simulink model "Pippo_sim"  (R2022b)
settings: Solver=ode1  StartTime=0.0  StopTime=inf  FixedStep=0.002  RelTol=1e-3  EnableMultiTasking=on
PostLoadFcn:
  | qc_set_target_type(getConfigSet(bdroot, 'QUARC Default Target Configuration'));
undefined symbols (not defined in the file or in its folder): HIL, qc_get_step_size
libraries: quarc_library x21, simulink_extras x7, simulink x6
settings Model: SimulationMode=external  ExtModeTrigDuration=10000  Creator=CFulford  LastModifiedBy=Utente
settings SolverCC: AlgebraicLoopSolver=TrustRegion  PositivePriorityOrder=on
settings DataIOCC: LimitDataPoints=on  SaveFormat=Array  SignalLoggingSaveFormat=ModelDataLogs  ReturnWorkspaceOutputs=off
settings OptimizationCC: ExpressionDepthLimit=2147483647  InitFltsAndDblsToZero=on
settings DebuggingCC: SaveWithParameterizedLinksMsg=none  UnderspecifiedInitializationDetection=Classic  MergeDetectMultiDrivingBlocksExec=none  SolverPrmCheckMsg=warning  MultiTaskDSMMsg=warning  MultiTaskCondExecSysMsg=none  FcnCallInpInsideContextMsg=warning  UnconnectedInputMsg=warning  UnconnectedOutputMsg=warning  UnconnectedLineMsg=warning  StateNameClashWarn=warning  SFUnexpectedBacktrackingDiag=warning  SFNoUnconditionalDefaultTransitionDiag=warning  SFExecutionAtInitializationDiag=none  SFMachineParentedDataDiag=warning  ArithmeticOperatorsInVariantConditions=warning
settings ModelReferenceCC: EnableRefExpFcnMdlSchedulingChecks=on  PropagateSignalLabelsOutOfModel=off
settings SFSimCC: SimUseLocalCustomCode=off  CustomCodeUndefinedFunction=UseInterfaceOnly
settings RTWCC: Description=QUARC Win64 Target Using Toolchain  SystemTargetFile=quarc_win64.tlc  TemplateMakefile=quarc_default_tmf  RTWUseLocalCustomCode=off  Toolchain=QUARC win64 | nmake (64-bit Windows)  BuildConfiguration=Faster Runs
settings CodeAppCC: StateflowObjectComments=on
settings STFCustomTargetCC: ConcurrentExecutionCompliant=on  GRTInterface=on  UseToolchainInfoCompliant=on  SystemTargetFile=quarc_win64.tlc
settings GRTTargetCC: TargetLangStandard=C89/C90 (ANSI)  ParMdlRefBuildCompliant=off  CompOptLevelCompliant=off  CombineOutputUpdateFcns=off  MatFileLogging=off  CPPClassGenCompliant=off  GRTInterface=on  ExtMode=on  ExtModeMexFile=quarc_comm
settings ConfigComp: CovMetricSettings=dw  CovSaveCumulativeToWorkspaceVar=on  CovSaveSingleToWorkspaceVar=on  CovExternalEMLEnable=off  CovSFcnEnable=off

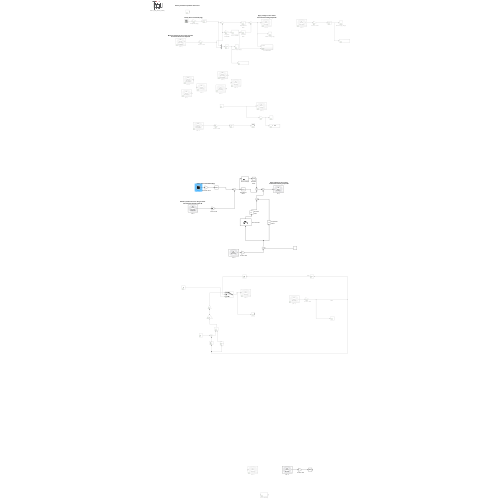
[thumbnail: Simulink's stored preview of the top-level diagram]
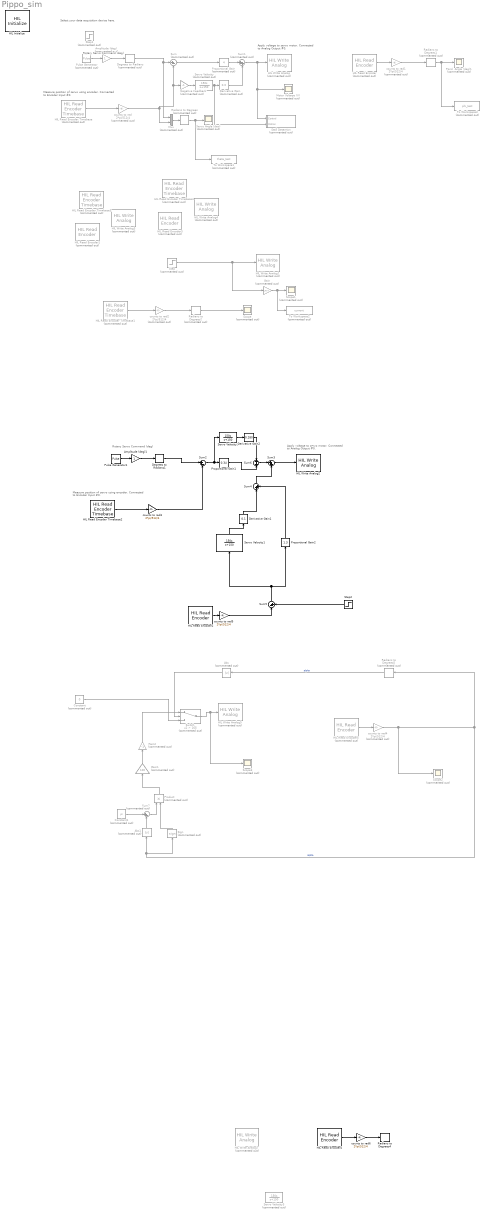
== system Pippo_sim ==
  note: Apply voltage to servo motor.
      | Connected to Analog Output #0.
  note: Measure position of servo using encoder.
      | Connected to Encoder Input #0.
  note: Select your data acquisition device here.
  note: Rotary Servo Command (deg)
  note: Measure position of servo using encoder.
      | Connected to Encoder Input #0.
  note: Rotary Servo Command (deg)
  note: Apply voltage to servo motor.
      | Connected to Analog Output #0.
  Abs : Abs  Commented=on  SaturateOnIntegerOverflow=off
  Abs1 : Abs  Commented=on  SaturateOnIntegerOverflow=off
  Amplitude (deg) : Gain  Commented=on
  Amplitude (deg)1 : Gain
  Constant : Constant  Commented=on  Value=0
  Constant1 : Constant  Commented=on  Value=pi
  Degrees to Radians : simulink_extras/Transformations/Degrees to Radians  Commented=on
  Degrees to Radians1 : simulink_extras/Transformations/Degrees to Radians
  Derivative Gain : simulink/Math Operations/Slider Gain  Commented=on  gain=0.0  low=0  high=0.5
  Derivative Gain1 : simulink/Math Operations/Slider Gain  gain=0.1  low=0  high=0.5
  Derivative Gain2 : simulink/Math Operations/Slider Gain  gain=0.280  low=0  high=0.5
  Gain : Gain  Commented=on  Gain=1/8.4
  Gain1 : Gain  Commented=on  Gain=100
  Gain2 : Gain  Commented=on  Gain=-1
  HIL Initialize : quarc_library/Data Acquisition/Generic/Configuration/HIL Initialize  Priority=-99  object_name=HIL-1  board_type=qube_servo2_usb  board_number=0  board_options=""  exclusive=off  active=off  hardware_clocks=[0]  clock_modes=[]  initial_clock_frequencies=[]  set_clock_params_at_start=off  set_clock_params_at_switch_in=off  set_clock_frequencies_at_start=off  set_clock_frequencies_at_switch_in=off  analog_input_channels=[0]  analog_input_configurations=[]  analog_input_maximums=3  analog_input_minimums=-3  set_analog_input_params_at_start=off  set_analog_input_params_at_switch_in=off  analog_output_channels=[0]  analog_output_maximums=15  analog_output_minimums=-15  initial_analog_outputs=[0]  final_analog_outputs=[0]  watchdog_analog_outputs=0  set_analog_output_params_at_start=off  set_analog_output_params_at_switch_in=off  set_analog_outputs_at_start=on  set_analog_outputs_at_switch_in=off  set_analog_outputs_at_terminate=on  set_analog_outputs_at_switch_out=off  set_analog_outputs_on_watchdog=on  digital_input_channels=[]  digital_output_channels=[0]  digital_output_configuration=[]  initial_digital_outputs=[1]  final_digital_outputs=[0]  watchdog_digital_outputs=[0]  set_digital_output_params_at_start=off  set_digital_output_params_at_switch_in=off  set_digital_outputs_at_start=on  set_digital_outputs_at_switch_in=off  set_digital_outputs_at_terminate=on  set_digital_outputs_at_switch_out=off  set_digital_outputs_on_watchdog=on  encoder_channels=[0:1]  quadrature=[4]  encoder_filter_frequency=[]  initial_encoder_counts=[0]  set_encoder_params_at_start=off  set_encoder_params_at_switch_in=off  set_encoder_counts_at_start=on  set_encoder_counts_at_switch_in=off  pwm_channels=[]  pwm_modes=[]  pwm_frequency=[]  pwm_configuration=[]  pwm_alignment=[]  pwm_polarity=[]  pwm_leading_deadband=[]  pwm_trailing_deadband=[]  initial_pwm_outputs=[]  final_pwm_outputs=[]  watchdog_pwm_outputs=[]  set_pwm_params_at_start=off  set_pwm_params_at_switch_in=off  set_pwm_outputs_at_start=off  set_pwm_outputs_at_switch_in=off  set_pwm_outputs_at_terminate=off  set_pwm_outputs_at_switch_out=off  set_pwm_outputs_on_watchdog=off  other_output_channels=[11000:11002]  initial_other_outputs=[0 1 0]  final_other_outputs=[1 0 0]  watchdog_other_outputs=[0 0 1]  set_other_outputs_at_start=on  set_other_outputs_at_switch_in=off  set_other_outputs_at_terminate=on  set_other_outputs_at_switch_out=off  set_other_outputs_on_watchdog=on
  HIL Read Encoder{,1,3,5} (4 alike) : quarc_library/Data Acquisition/Generic/Immediate I//O/HIL Read Encoder  Commented=on  object_name=HIL-1  channels=[1]  sample_time=qc_get_step_size  active=on  vector_output=off  data_type_mode=Inherit via back propagation  data_type=double
  HIL Read Encoder Timebase{,1,3..4} (4 alike) : quarc_library/Data Acquisition/Generic/Timebases/HIL Read Encoder Timebase  Commented=on  object_name=HIL-1  clock=0  channels=0  active=on  vector_output=off  data_type_mode=Inherit via back propagation  data_type=double  overflow_mode=Error on overflow  samples_in_buffer=max(ceil(1/qc_get_step_size), 1)
  HIL Read Encoder Timebase2 : quarc_library/Data Acquisition/Generic/Timebases/HIL Read Encoder Timebase  object_name=HIL-1  clock=0  channels=0  active=on  vector_output=off  data_type_mode=Inherit via back propagation  data_type=double  overflow_mode=Error on overflow  samples_in_buffer=max(ceil(1/qc_get_step_size), 1)
  HIL Read Encoder2 : quarc_library/Data Acquisition/Generic/Immediate I//O/HIL Read Encoder  object_name=HIL-1  channels=[1]  sample_time=qc_get_step_size  active=on  vector_output=off  data_type_mode=Inherit via back propagation  data_type=double
  HIL Read Encoder4 : quarc_library/Data Acquisition/Generic/Immediate I//O/HIL Read Encoder  object_name=HIL-1  channels=[1]  sample_time=qc_get_step_size  active=on  vector_output=off  data_type_mode=Inherit via back propagation  data_type=double
  HIL Write Analog{,1,3..5,7} (6 alike) : quarc_library/Data Acquisition/Generic/Immediate I//O/HIL Write Analog  Commented=on  object_name=HIL-1  channels=0  sample_time=-1  active=off  vector_input=off
  HIL Write Analog2 : quarc_library/Data Acquisition/Generic/Immediate I//O/HIL Write Analog  object_name=HIL-1  channels=0  sample_time=-1  active=off  vector_input=off
  Motor Voltage (V) : Scope  Commented=on
  Mux : Mux  Commented=on  Inputs=2
  Negative Feedback : Gain  Commented=on  Gain=-1
  Pend  Angle (deg)1 : Scope  Commented=on
  Product : Product  Commented=on
  Proportional Gain : simulink/Math Operations/Slider Gain  Commented=on  gain=4  low=0  high=10
  Proportional Gain1 : simulink/Math Operations/Slider Gain  gain=0.34  low=0  high=10
  Proportional Gain2 : simulink/Math Operations/Slider Gain  gain=1.3  low=0  high=10
  Pulse Generator : DiscretePulseGenerator  Commented=on  PulseType=Time based  Amplitude=90  Period=10  PulseWidth=50
  Pulse Generator1 : DiscretePulseGenerator  PulseType=Time based  Amplitude=0  Period=10  PulseWidth=50
  Radians to Degrees{,1..2,5} (4 alike) : simulink_extras/Transformations/Radians to Degrees  Commented=on
  Radians to Degrees4 : simulink_extras/Transformations/Radians to Degrees
  Scope{,1..3} (4 alike) : Scope  Commented=on
  Servo Angle (deg) : Scope  Commented=on
  Servo Velocity : TransferFcn  Commented=on  Numerator=[150 0]  Denominator=[1 150]
  Servo Velocity1 : TransferFcn  Numerator=[150 0]  Denominator=[1 150]
  Servo Velocity2 : TransferFcn  Numerator=[150 0]  Denominator=[1 150]
  Servo Velocity3 : TransferFcn  Commented=on  Numerator=[150 0]  Denominator=[1 150]
  Sign : Signum  Commented=on
  Stall Detection : Subsystem  Commented=on
  Step : Step  Commented=on  SampleTime=0
  Step1 : Step  Commented=on  After=45  SampleTime=0
  Step2 : Step  Time=0  After=0  SampleTime=0
  Sum : Sum  Commented=on  Inputs=|+-
  Sum1 : Sum  Commented=on  Inputs=|++
  Sum2 : Sum  Inputs=|+-
  Sum3 : Sum  Inputs=|++
  Sum4 : Sum  Inputs=|++
  Sum5 : Sum  Inputs=|-+
  Sum6 : Sum
  Sum7 : Sum  Commented=on  Inputs=|+-
  Switch : Switch  Commented=on  Criteria=u2 > Threshold  Threshold=165  SaturateOnIntegerOverflow=off  InputSameDT=off
  To Workspace1 : ToWorkspace  Commented=on  VariableName=theta_test  SaveFormat=Structure With Time  SampleTime=-1
  To Workspace2 : ToWorkspace  Commented=on  VariableName=current  SaveFormat=Structure With Time  SampleTime=-1
  To Workspace3 : ToWorkspace  Commented=on  VariableName=phi_test  SaveFormat=Structure With Time  SampleTime=-1
  counts to rad{,1..2,4} (4 alike) : Gain  Commented=on  Gain=2*pi/512/4
  counts to rad3 : Gain  Gain=2*pi/512/4
  counts to rad5 : Gain  Gain=2*pi/512/4
  counts to rad6 : Gain  Gain=2*pi/512/4
  wires:
  Sum1/1 -> HIL Write Analog/1, Stall Detection/1(Control), Motor Voltage (V)/1
  Sum/1 -> Proportional Gain/1
  counts to rad/1 -> Sum/2, Negative Feedback/1, Mux/2
  Proportional Gain/1 -> Sum1/1
  Servo Velocity/1 -> Stall Detection/2(Motion), Derivative Gain/1
  Derivative Gain/1 -> Sum1/2
  Degrees to Radians/1 -> Mux/1, Sum/1
  Negative Feedback/1 -> Servo Velocity/1
  Mux/1 -> Radians to Degrees/1
  Radians to Degrees/1 -> To Workspace1/1, Servo Angle (deg)/1
  HIL Read Encoder/1 -> counts to rad1/1
  Radians to Degrees1/1 -> To Workspace3/1, Pend  Angle (deg)1/1
  counts to rad1/1 -> Radians to Degrees1/1
  Amplitude (deg)/1 -> Degrees to Radians/1
  Pulse Generator/1 -> Amplitude (deg)/1
  HIL Read Encoder Timebase/1 -> counts to rad/1
  Step/1 -> Gain/1, HIL Write Analog1/1
  HIL Read Encoder Timebase1/1 -> counts to rad2/1
  counts to rad2/1 -> Radians to Degrees2/1
  Gain/1 -> To Workspace2/1, Scope1/1
  Radians to Degrees2/1 -> Scope/1
  Pulse Generator1/1 -> Amplitude (deg)1/1
  Amplitude (deg)1/1 -> Degrees to Radians1/1
  Proportional Gain1/1 -> Sum6/2
  Sum3/1 -> HIL Write Analog2/1
  counts to rad3/1 -> Sum2/2
  HIL Read Encoder Timebase2/1 -> counts to rad3/1
  Sum5/1 -> Servo Velocity1/1, Proportional Gain2/1
  HIL Read Encoder2/1 -> counts to rad5/1
  Proportional Gain2/1 -> Sum4/2
  Servo Velocity1/1 -> Derivative Gain1/1
  Derivative Gain1/1 -> Sum4/1
  counts to rad5/1 -> Sum5/1
  Step2/1 -> Sum5/2
  Degrees to Radians1/1 -> Sum2/1
  Sum2/1 -> Servo Velocity2/1, Proportional Gain1/1
  Servo Velocity2/1 -> Derivative Gain2/1
  Sum6/1 -> Sum3/1
  Sum4/1 -> Sum3/2
  Derivative Gain2/1 -> Sum6/1
  counts to rad4/1 -> Sign/1, Abs1/1, Radians to Degrees5/1, Scope2/1  "alpha"
  Switch/1 -> HIL Write Analog5/1, Scope3/1
  Abs/1 -> Switch/2
  Constant/1 -> Switch/3
  Constant1/1 -> Sum7/1
  Abs1/1 -> Sum7/2
  Sum7/1 -> Product/1
  Sign/1 -> Product/2
  Product/1 -> Gain1/1
  Gain1/1 -> Gain2/1
  HIL Read Encoder5/1 -> counts to rad4/1
  Gain2/1 -> Switch/1
  HIL Read Encoder4/1 -> counts to rad6/1
  counts to rad6/1 -> Radians to Degrees4/1
  Radians to Degrees5/1 -> Abs/1  "alpha"

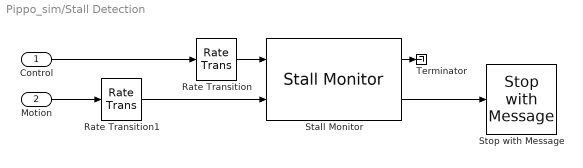
== system Pippo_sim/Stall Detection ==
  Control : Inport
  Motion : Inport  Port=2
  Rate Transition : RateTransition
  Rate Transition1 : RateTransition
  Stall Monitor : quarc_library/Discrete/Stall Monitor  control_threshold=5  motion_threshold=0.3  duration_s=20
      settings: SourceProductName=QUARC Targets
  Stop with Message : quarc_library/Sinks/Error Handling/Stop with Message  message_type=Fixed error message  message_icon=Error  message=Stall Detected! Please ensure that the DC motor is free to move and is functioning properly
  Terminator : Terminator
  wires:
  Control/1 -> Rate Transition/1
  Motion/1 -> Rate Transition1/1
  Stall Monitor/2 -> Stop with Message/1
  Stall Monitor/1 -> Terminator/1
  Rate Transition/1 -> Stall Monitor/1
  Rate Transition1/1 -> Stall Monitor/2
